simulink model "randomInputModel"  (R2017b)
settings: Solver=VariableStepAuto  StartTime=0.0  StopTime=500  RelTol=1e-3  EnableMultiTasking=on
settings Model: Creator=Asus  LastModifiedBy=root
settings DataIOCC: LimitDataPoints=on
settings OptimizationCC: LifeSpan=inf
settings DebuggingCC: AllowSymbolicDim=off  SFUnexpectedBacktrackingDiag=warning  SFNoUnconditionalDefaultTransitionDiag=warning  SFExecutionAtInitializationDiag=none
settings ModelReferenceCC: PropagateSignalLabelsOutOfModel=off
settings CodeAppCC: StateflowObjectComments=on
settings GRTTargetCC: TargetLangStandard=C89/C90 (ANSI)
settings ConfigComp: CovMetricSettings=dw  CovHtmlReporting=on  CovSaveCumulativeToWorkspaceVar=on  CovSaveSingleToWorkspaceVar=on  CovExternalEMLEnable=off

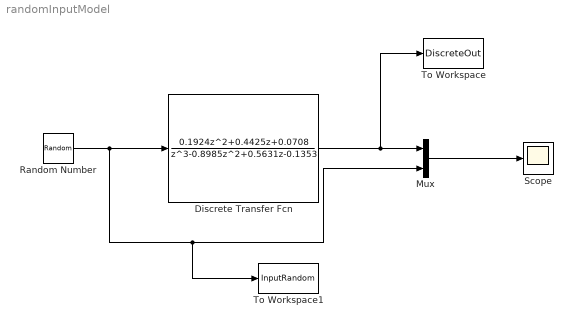
== system randomInputModel ==
  Discrete Transfer Fcn : DiscreteTransferFcn  Numerator=[0 0.1924 0.4425 0.0708]  Denominator=[1 -0.8985 0.5631 -0.1353]  SampleTime=1
  Mux : Mux  Inputs=2
  Random Number : RandomNumber  SampleTime=1
  Scope : Scope
  To Workspace : ToWorkspace  VariableName=DiscreteOut  SampleTime=1
  To Workspace1 : ToWorkspace  VariableName=InputRandom  SampleTime=1
  wires:
  Random Number/1 -> Discrete Transfer Fcn/1, To Workspace1/1, Mux/2
  Discrete Transfer Fcn/1 -> To Workspace/1, Mux/1
  Mux/1 -> Scope/1
